simulink library "ComputeNorm2D"  (R2014b)
settings: Solver=ode45  StartTime=0.0  StopTime=10.0  RelTol=1e-3
settings Model: Creator=Hp  LastModifiedBy=Hp

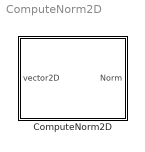
== system ComputeNorm2D ==
  ComputeNorm2D : Subsystem

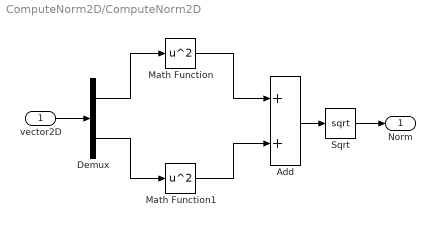
== system ComputeNorm2D/ComputeNorm2D ==
  vector2D : Inport
  Add : Sum
  Demux : Demux  Outputs=2
  Math Function : Math  Operator=square  SaturateOnIntegerOverflow=on
  Math Function1 : Math  Operator=square  SaturateOnIntegerOverflow=on
  Sqrt : Sqrt  SaturateOnIntegerOverflow=on
  Norm : Outport
  wires:
  Demux/2 -> Math Function1/1
  Math Function/1 -> Add/1
  Demux/1 -> Math Function/1
  Math Function1/1 -> Add/2
  Add/1 -> Sqrt/1
  Sqrt/1 -> Norm/1
  vector2D/1 -> Demux/1
